simulink model "TV2016_CAN"  (Simulink 8.5)
settings: Solver=ode1  StartTime=0.0  StopTime=inf  FixedStep=0.001  RelTol=1e-3
PreLoadFcn:
  | FSE_Parameters
values from neighbouring files (symbols this model uses):
  car_params = Simulink_Car_params    [TV2016_parameters.m]
  i_Diff = 15.47    [TV2016_parameters.m]
  Kp = 1    [TV2016_parameters.m]
  settings = Simulink_Settings    [TV2016_parameters.m]
  SpdC_BCC = 0    [TV2016_parameters.m]
  Speed_Neg_sat = -21    [TV2016_parameters.m]
  Speed_Pos_sat = 21    [TV2016_parameters.m]
  Tn_n = 0    [TV2016_parameters.m]
  Use_Joystick = 1    [TV2016_parameters.m]
undefined symbols (not defined in the file or in its folder): canChannel
libraries: CarMaker4SL x139, simulink x18, canmsglib x10, simulink_extras x7, canlib x5, sldrtlib x1
(part 1 of 4)
settings Model: Creator=fh  LastModifiedBy=Will
settings SolverCC: EnableConcurrentExecution=on  InsertRTBMode=Always
settings DataIOCC: SignalLoggingName=sigsOut
settings OptimizationCC: BlockReduction=off  OptimizeBlockIOStorage=off  BufferReuse=off  GlobalBufferReuse=off  ExpressionFolding=off  LocalBlockOutputs=off  InitFltsAndDblsToZero=on
settings DebuggingCC: SaveWithParameterizedLinksMsg=none  SignalResolutionControl=TryResolveAllWithWarning  MultiTaskDSMMsg=warning  MultiTaskCondExecSysMsg=none  FcnCallInpInsideContextMsg=UseLocalSettings  BusObjectLabelMismatch=error
settings HardwareCC: ProdBitPerLong=64  ProdBitPerPointer=64  ProdIntDivRoundTo=Zero  ProdEndianess=LittleEndian  ProdWordSize=64  ProdHWDeviceType=Intel->x86-64  TargetBitPerLong=64  TargetBitPerPointer=64  TargetIntDivRoundTo=Zero  TargetEndianess=LittleEndian  TargetWordSize=64  TargetHWDeviceType=Intel->x86-64
settings SFSimCC: SimCtrlC=off
settings RTWCC: SystemTargetFile=rtwin.tlc  TemplateMakefile=rtwin.tmf  Description=Simulink Desktop Real-Time  Toolchain=LCC-win64 v2.4.1 | gmake (64-bit Windows)  BuildConfiguration=Faster Runs  RTWCompilerOptimization=on  CheckMdlBeforeBuild=Warning
settings CodeAppCC: MaxIdLength=95
settings RTWinTargetCC: TargetPreCompLibLocation=D:\Program Files\MATLAB\R2015a\toolbox\sldrt\lib\win64

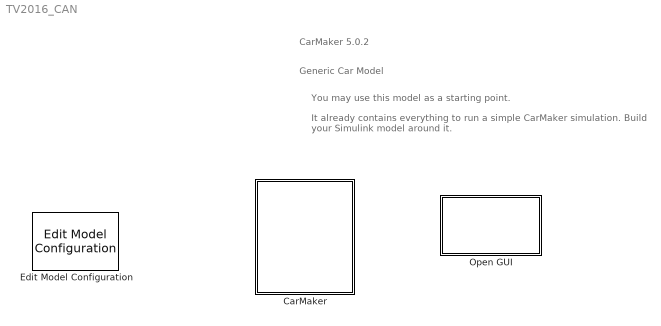
== system TV2016_CAN ==
  note: Generic Car Model
  note: You may use this model as a starting point.
  note: It already contains everything to run a simple CarMaker simulation.
      | Build your Simulink model around it.
  note: CarMaker 5.0.2
  CarMaker : Subsystem  TreatAsAtomicUnit=on
      mask Display: image(imread('CarMaker4SLss.bmp'));
  Edit Model Configuration : CarMaker4SL/Edit Model Configuration
  Open GUI : Subsystem  LoadFcn=if ~length(which('cmcmd')), cmenv; end
      settings: OpenFcn=cmblockmagic('gui_fix_display'); CM_Simulink
      mask Display: image(imread('CarMakerGUI.bmp'));

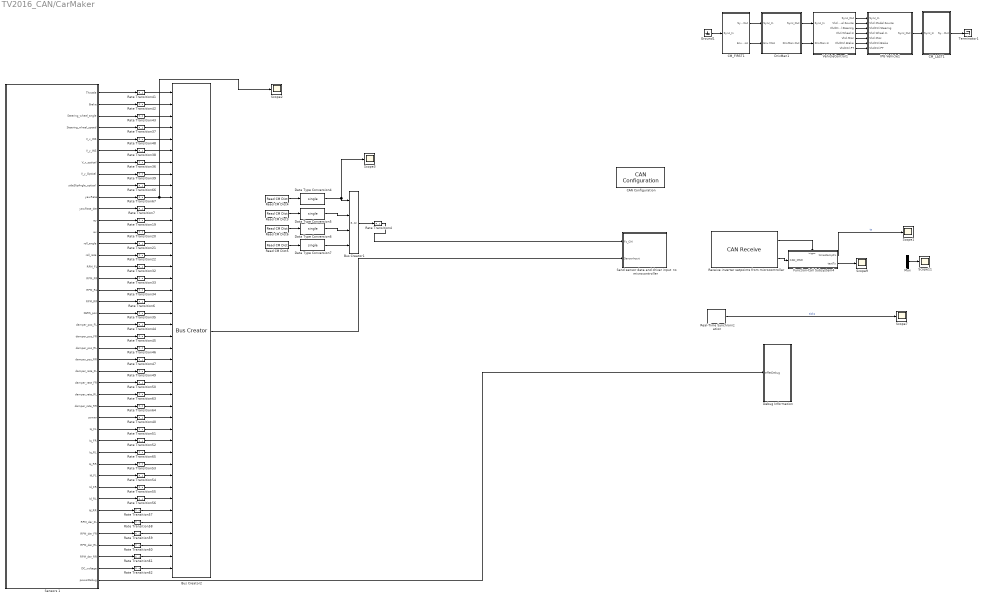
== system TV2016_CAN/CarMaker ==
  Bus Creator1 : BusCreator  OutDataTypeStr=Bus: normalForces  NonVirtualBus=on
      settings: InheritFromInputs=off
  Bus Creator2 : BusCreator  Inputs=42  OutDataTypeStr=Bus: SensorInputs  NonVirtualBus=on
      settings: InheritFromInputs=off
  CAN Configuration : canlib/CAN Configuration  BlockHandle=4619.0087  DeviceMenu=(none)  Device=PEAK-System PCAN-USB (PCAN_USBBUS1)  ObjConstructor=canChannel('PEAK-System', 'PCAN_USBBUS1')  BusSpeed=1000000  EnableBitParameters=off  SJW=NaN  TSEG1=NaN  TSEG2=NaN  NSamples=NaN  AckMode=Normal
  CM_FIRST1 : Subsystem
  CM_LAST1 : Subsystem
  Data Type Conversion{4..7} (4 alike) : DataTypeConversion  OutDataTypeStr=single
  "Debug Information " : Subsystem
  DrivMan1 : Subsystem
  Function-Call Subsystem4 : Subsystem  TreatAsAtomicUnit=on
  Ground1 : Ground
  IPG Vehicle1 : Subsystem  TreatAsAtomicUnit=on
  Mux : Mux  Inputs=2
  Rate Transition{4,6..7,19..22,32..67} (43 alike) : RateTransition  OutPortSampleTime=settings.sensor_sampling_time
  Read CM Dict3 : CarMaker4SL/Read CM Dict  xname=Vhcl.FR.Fz  xsync=off
  Read CM Dict4 : CarMaker4SL/Read CM Dict  xname=Vhcl.FL.Fz  xsync=off
  Read CM Dict5 : CarMaker4SL/Read CM Dict  xname=Vhcl.RR.Fz  xsync=off
  Read CM Dict6 : CarMaker4SL/Read CM Dict  xname=Vhcl.RL.Fz  xsync=off
  Real-Time Synchronization : sldrtlib/Real-Time Synchronization  SampleTime=0.001  MaxMissedTicks=100000  ShowMissedTicks=on  YieldWhenWaiting=off
  Receive inverter setpoints from microcontroller : canlib/CAN Receive  BlockHandle=12566.0002  DeviceMenu=(none)  Device=PEAK-System PCAN-USB (PCAN_USBBUS1)  ObjConstructor=canChannel('PEAK-System', 'PCAN_USBBUS1')  EnableStandardIDsFilter=off  StandardIDs=[387,388,389,390,800]  EnableExtendedIDsFilter=off  ExtendedIDs=0  SampleTime=0.001  MsgsPerTimestep=all  StdIDsCombo=Allow only  ExtIDsCombo=Block all  InternalFilterUpdateStatus=on
  Scope{1..3,7,9,11} (6 alike) : Scope
      Scope1 settings: ShowLegends=on  TimeRange=2.184524711696869  YMin=-0.01  YMax=0.02  SaveName=ScopeData26
      Scope11 settings: ShowLegends=on  TimeRange=2.184524711696869  YMin=-0.01  YMax=0.02  SaveName=ScopeData25
      Scope2 settings: ShowLegends=on  TimeRange=9.572585353545549e-05  YMin=0  YMax=1000  SaveName=ScopeData45
      Scope3 settings: ShowLegends=on  TimeRange=9.572585353545549e-05  YMin=0  YMax=1000  SaveName=ScopeData51
      Scope7 settings: ShowLegends=on  TimeRange=9.572585353545549e-05  YMin=0  YMax=1000  SaveName=ScopeData14
      Scope9 settings: YMin=2  YMax=15  SaveName=ScopeData38  SampleInput=on  SampleTime=0.001
  "Send sensor data and driver input  to microcontroller " : Subsystem
  Sensors 1 : Subsystem  SystemSampleTime=settings.control_system_sample_time
  Terminator1 : Terminator
  VehicleControl1 : Subsystem
  wires:
  Read CM Dict3/1 -> Data Type Conversion5/1
  Read CM Dict4/1 -> Data Type Conversion4/1
  Read CM Dict5/1 -> Data Type Conversion7/1
  Read CM Dict6/1 -> Data Type Conversion6/1
  Data Type Conversion6/1 -> Bus Creator1/3
  Data Type Conversion7/1 -> Bus Creator1/4
  Data Type Conversion5/1 -> Bus Creator1/2
  Data Type Conversion4/1 -> Scope3/1, Bus Creator1/1
  Bus Creator1/1 -> Rate Transition4/1
  Rate Transition4/1 -> "Send sensor data and driver input  to microcontroller "/1(Fz_CM)
  Real-Time Synchronization/1 -> Scope7/1  "ticks"
  Receive inverter setpoints from microcontroller/2 -> Function-Call Subsystem4/1(CAN_MSG)
  Receive inverter setpoints from microcontroller/1 -> Function-Call Subsystem4/Trigger
  Function-Call Subsystem4/1(timestampFL) -> Scope1/1  "ts"
  Mux/1 -> Scope11/1
  Function-Call Subsystem4/2(testTs) -> Scope9/1
  Sensors 1/43(powerDebug) -> "Debug Information "/1(effetDebug)
  Bus Creator2/1 -> "Send sensor data and driver input  to microcontroller "/2(SensorInput)
  Sensors 1/40(RPM_der_RL) -> Rate Transition60/1
  Sensors 1/41(RPM_der_RR) -> Rate Transition61/1
  Sensors 1/39(RPM_der_FR) -> Rate Transition59/1
  Sensors 1/38(RPM_der_FL) -> Rate Transition58/1
  Sensors 1/37(Id_RR) -> Rate Transition57/1
  Sensors 1/4(Steering_wheel_speed) -> Rate Transition37/1
  Sensors 1/1("Throttle ") -> Rate Transition41/1
  Sensors 1/2("Brake ") -> Rate Transition42/1
  Sensors 1/3("Steering_wheel_angle ") -> Rate Transition43/1
  Sensors 1/5(V_x_INS) -> Rate Transition48/1
  Sensors 1/6(V_y_INS) -> Rate Transition38/1
  Sensors 1/7(V_x_optical) -> Rate Transition36/1
  Sensors 1/8(V_y_Optical) -> Rate Transition39/1
  Sensors 1/9(sideSlipAngle_optical) -> Rate Transition66/1
  Sensors 1/10(yawRate) -> Rate Transition67/1
  Sensors 1/12(ay) -> Rate Transition19/1
  Sensors 1/13("ax ") -> Rate Transition20/1
  Sensors 1/14(roll_angle) -> Rate Transition21/1
  Sensors 1/15(roll_rate) -> Rate Transition22/1
  Sensors 1/16(RPM_FL) -> Rate Transition32/1
  Sensors 1/17(RPM_FR) -> Rate Transition33/1
  Sensors 1/18(RPM_RL) -> Rate Transition34/1
  Sensors 1/19(RPM_RR) -> Rate Transition6/1
  Sensors 1/20(KERS_pos) -> Rate Transition35/1
  Sensors 1/21(damper_pos_FL) -> Rate Transition44/1
  Sensors 1/22(damper_pos_FR) -> Rate Transition45/1
  Sensors 1/23(damper_pos_RL) -> Rate Transition46/1
  Sensors 1/24(damper_pos_RR) -> Rate Transition47/1
  Sensors 1/25(damper_rate_FL) -> Rate Transition49/1
  Sensors 1/26(damper_rate_FR) -> Rate Transition50/1
  Sensors 1/27(damper_rate_RL) -> Rate Transition63/1
  Sensors 1/28(damper_rate_RR) -> Rate Transition64/1
  Sensors 1/29(power) -> Rate Transition40/1
  Sensors 1/30(Iq_FL) -> Rate Transition51/1
  Sensors 1/31(Iq_FR) -> Rate Transition52/1
  Sensors 1/32(Iq_RL) -> Rate Transition65/1
  Sensors 1/33(Iq_RR) -> Rate Transition53/1
  Sensors 1/34(Id_FL) -> Rate Transition54/1
  Sensors 1/35(Id_FR) -> Rate Transition55/1
  Sensors 1/36(Id_RL) -> Rate Transition56/1
  Sensors 1/11(yawRate_der) -> Rate Transition7/1
  Sensors 1/42(DC_voltage) -> Rate Transition62/1
  Rate Transition62/1 -> Bus Creator2/42
  Rate Transition6/1 -> Bus Creator2/19
  Rate Transition7/1 -> Bus Creator2/11
  Rate Transition19/1 -> Bus Creator2/12
  Rate Transition20/1 -> Bus Creator2/13
  Rate Transition21/1 -> Bus Creator2/14
  Rate Transition22/1 -> Bus Creator2/15
  Rate Transition32/1 -> Bus Creator2/16
  Rate Transition33/1 -> Bus Creator2/17
  Rate Transition34/1 -> Bus Creator2/18
  Rate Transition35/1 -> Bus Creator2/20
  Rate Transition36/1 -> Bus Creator2/7
  Rate Transition37/1 -> Bus Creator2/4
  Rate Transition38/1 -> Bus Creator2/6
  Rate Transition39/1 -> Bus Creator2/8
  Rate Transition40/1 -> Bus Creator2/29
  Rate Transition41/1 -> Bus Creator2/1
  Rate Transition42/1 -> Bus Creator2/2
  Rate Transition43/1 -> Bus Creator2/3
  Rate Transition44/1 -> Bus Creator2/21
  Rate Transition45/1 -> Bus Creator2/22
  Rate Transition46/1 -> Bus Creator2/23
  Rate Transition47/1 -> Bus Creator2/24
  Rate Transition48/1 -> Bus Creator2/5
  Rate Transition49/1 -> Bus Creator2/25
  Rate Transition50/1 -> Bus Creator2/26
  Rate Transition51/1 -> Bus Creator2/30
  Rate Transition52/1 -> Bus Creator2/31
  Rate Transition53/1 -> Bus Creator2/33
  Rate Transition54/1 -> Bus Creator2/34
  Rate Transition55/1 -> Bus Creator2/35
  Rate Transition56/1 -> Bus Creator2/36
  Rate Transition63/1 -> Bus Creator2/27
  Rate Transition64/1 -> Bus Creator2/28
  Rate Transition65/1 -> Bus Creator2/32
  Rate Transition66/1 -> Bus Creator2/9
  Rate Transition67/1 -> Scope2/1, Bus Creator2/10
  Rate Transition57/1 -> Bus Creator2/37
  Rate Transition58/1 -> Bus Creator2/38
  Rate Transition59/1 -> Bus Creator2/39
  Rate Transition60/1 -> Bus Creator2/40
  Rate Transition61/1 -> Bus Creator2/41
  DrivMan1/2(DrivMan.Out) -> VehicleControl1/2(DrivMan.In)
  DrivMan1/1(Sync_Out) -> VehicleControl1/1(Sync_In)
  CM_FIRST1/2(Env.Misc) -> DrivMan1/2(Env.Misc)
  CM_FIRST1/1(Sync_Out) -> DrivMan1/1(Sync_In)
  CM_LAST1/1(Sync_Out) -> Terminator1/1
  IPG Vehicle1/1(Sync_Out) -> CM_LAST1/1(Sync_In)
  VehicleControl1/1(Sync_Out) -> IPG Vehicle1/1(Sync_In)
  VehicleControl1/3(VhclCtrl.Steering) -> IPG Vehicle1/3(VhclCtrl.Steering)
  VehicleControl1/4(Vhcl.Wheel.In) -> IPG Vehicle1/4(Vhcl.Wheel.In)
  VehicleControl1/5(Vhcl.Misc) -> IPG Vehicle1/5(Vhcl.Misc)
  VehicleControl1/6(VhclCtrl.Brake) -> IPG Vehicle1/6(VhclCtrl.Brake)
  VehicleControl1/7(VhclCtrl.PT) -> IPG Vehicle1/7(VhclCtrl.PT)
  VehicleControl1/2(Vhcl.Model.Source) -> IPG Vehicle1/2(Vhcl.Model.Source)
  Ground1/1 -> CM_FIRST1/1(Sync_In)

== system TV2016_CAN/Open GUI ==
  S-Function : S-Function  FunctionName=cm_gui

== system TV2016_CAN/CarMaker/CM_FIRST1 ==
  Sync_In : Inport
  Bus Creator1 : BusCreator  Inputs=9
  Demux : Demux  Outputs=9
  Environment : S-Function  FunctionName=CM_Sfun  Parameters='Environment'
  IoIn : S-Function  FunctionName=CM_Sfun  Parameters='IoIn'
  Sync_Out : Outport
  Env.Misc : Outport  Port=2
  wires:
  Bus Creator1/1 -> Env.Misc/1
  Environment/2 -> Demux/1
  Demux/4 -> Bus Creator1/4  "Env AirHumidity"
  Demux/3 -> Bus Creator1/3  "Env AirPressure"
  Demux/2 -> Bus Creator1/2  "Env AirDensity"
  Demux/1 -> Bus Creator1/1  "Env Temperature"
  Environment/1 -> Sync_Out/1
  IoIn/1 -> Environment/1
  Sync_In/1 -> IoIn/1
  Demux/5 -> Bus Creator1/5  "Env Time"
  Demux/6 -> Bus Creator1/6  "Env SolarRadiation"
  Demux/7 -> Bus Creator1/7  "Env WindVel_tot x"
  Demux/8 -> Bus Creator1/8  "Env WindVel_tot y"
  Demux/9 -> Bus Creator1/9  "Env WindVel_tot z"

== system TV2016_CAN/CarMaker/CM_LAST1 ==
  Sync_In : Inport
  CM_User : S-Function  FunctionName=CM_Sfun  Parameters='CM_User'
  IoOut : S-Function  FunctionName=CM_Sfun  Parameters='IoOut'
  Sync_Out : Outport
  wires:
  IoOut/1 -> Sync_Out/1
  CM_User/1 -> IoOut/1
  Sync_In/1 -> CM_User/1

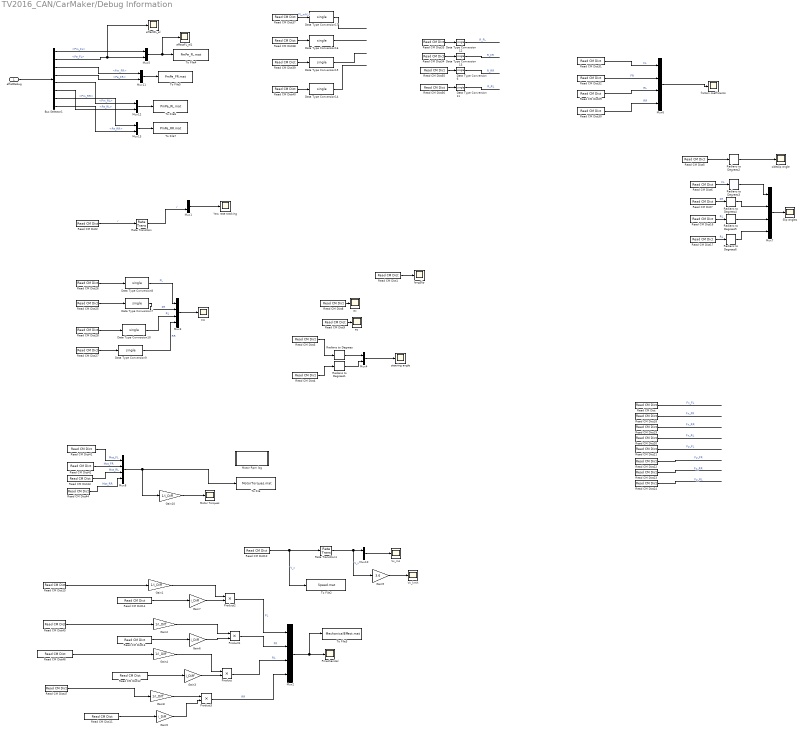
== system TV2016_CAN/CarMaker/Debug Information  ==
  effetDebug : Inport
  Bus Selector1 : BusSelector  OutputSignals=Pm_FL,Pe_FL,Pm_FR,Pe_FR,Pm_RL,Pe_RL,Pm_RR,Pe_RR
  Data Type Conversion{6..17} (12 alike) : DataTypeConversion  OutDataTypeStr=single
  Fzi : Scope
      settings: ShowLegends=on  TimeRange=18.75514233997038  YMin=0  YMax=1400  SaveName=ScopeData21
  Gain{1..2,4,8,10} (5 alike) : Gain  Gain=1/i_Diff
  Gain{3,5..7} (4 alike) : Gain  Gain=i_Diff
  Gain9 : Gain  Gain=3.6
  "Motor Rpm log  " : Subsystem
  "Motor Torques " : Scope
      settings: ShowLegends=on  TimeRange=0.2362659824329911  YMin=0.3167539267015711  YMax=0.6151832460732987  SaveName=ScopeData8
  Mux{1,4..5,10..13} (7 alike) : Mux  Inputs=2
  Mux{2..3,6..8} (5 alike) : Mux
  Pmechanical : Scope
      settings: TimeRange=6  YMin=-25  YMax=275  SaveName=ScopeData20
  Product{,1..3} (4 alike) : Product
  Radians to Degrees{,1..6} (7 alike) : simulink_extras/Transformations/Radians to Degrees
  Rate Transition : RateTransition  OutPortSampleTime=settings.control_system_sample_time
  Rate Transition1 : RateTransition  OutPortSampleTime=settings.control_system_sample_time
  Read CM Dict : CarMaker4SL/Read CM Dict  xname=Vhcl.FL.Fx  xsync=off
  Read CM Dict1 : CarMaker4SL/Read CM Dict  xname=Car.LongSlipRL  xsync=off
  Read CM Dict10 : CarMaker4SL/Read CM Dict  xname=Car.vx  xsync=off
  Read CM Dict11 : CarMaker4SL/Read CM Dict  xname=Car.WheelSpd_RR  xsync=off
  Read CM Dict12 : CarMaker4SL/Read CM Dict  xname=Car.WheelSpd_RL  xsync=off
  Read CM Dict13 : CarMaker4SL/Read CM Dict  xname=Car.WheelSpd_FR  xsync=off
  Read CM Dict14 : CarMaker4SL/Read CM Dict  xname=Car.WheelSpd_FL  xsync=off
  Read CM Dict15 : CarMaker4SL/Read CM Dict  xname=PT.WFL.Trq_Drive  xsync=off
  Read CM Dict16 : CarMaker4SL/Read CM Dict  xname=Car.SlipAngleRL  xsync=off
  Read CM Dict17 : CarMaker4SL/Read CM Dict  xname=Car.SlipAngleRR  xsync=off
  Read CM Dict18 : CarMaker4SL/Read CM Dict  xname=Vhcl.FR.Fx  xsync=off
  Read CM Dict19 : CarMaker4SL/Read CM Dict  xname=Vhcl.RR.Fx  xsync=off
  Read CM Dict2 : CarMaker4SL/Read CM Dict  xname=Car.YawRate  xsync=off
  Read CM Dict20 : CarMaker4SL/Read CM Dict  xname=Vhcl.RL.Fx  xsync=off
  Read CM Dict21 : CarMaker4SL/Read CM Dict  xname=Vhcl.FL.Fy  xsync=off
  Read CM Dict22 : CarMaker4SL/Read CM Dict  xname=Vhcl.FR.Fy  xsync=off
  Read CM Dict23 : CarMaker4SL/Read CM Dict  xname=Vhcl.RR.Fy  xsync=off
  Read CM Dict24 : CarMaker4SL/Read CM Dict  xname=Vhcl.RL.Fy  xsync=off
  Read CM Dict25 : CarMaker4SL/Read CM Dict  xname=Vhcl.FR.Fz  xsync=off
  Read CM Dict26 : CarMaker4SL/Read CM Dict  xname=Vhcl.FL.Fz  xsync=off
  Read CM Dict27 : CarMaker4SL/Read CM Dict  xname=Vhcl.RR.Fz  xsync=off
  Read CM Dict28 : CarMaker4SL/Read CM Dict  xname=Vhcl.RL.Fz  xsync=off
  Read CM Dict29 : CarMaker4SL/Read CM Dict  xname=Car.muRoadRL  xsync=off
  Read CM Dict3 : CarMaker4SL/Read CM Dict  xname=Car.CFR.rz  xsync=off
  Read CM Dict30 : CarMaker4SL/Read CM Dict  xname=Car.muRoadRR  xsync=off
  Read CM Dict31 : CarMaker4SL/Read CM Dict  xname=Car.muRoadFL  xsync=off
  Read CM Dict32 : CarMaker4SL/Read CM Dict  xname=Car.muRoadFR  xsync=off
  Read CM Dict33 : CarMaker4SL/Read CM Dict  xname=Car.WFL.Radius  xsync=off
  Read CM Dict34 : CarMaker4SL/Read CM Dict  xname=Car.WFR.Radius  xsync=off
  Read CM Dict35 : CarMaker4SL/Read CM Dict  xname=Car.WRR.Radius  xsync=off
  Read CM Dict36 : CarMaker4SL/Read CM Dict  xname=Car.WRL.Radius  xsync=off
  Read CM Dict37 : CarMaker4SL/Read CM Dict  xname=Car.vFL  xsync=off
  Read CM Dict38 : CarMaker4SL/Read CM Dict  xname=Car.vFR  xsync=off
  Read CM Dict39 : CarMaker4SL/Read CM Dict  xname=Car.vRR  xsync=off
  Read CM Dict4 : CarMaker4SL/Read CM Dict  xname=Car.CFL.rz  xsync=off
  Read CM Dict40 : CarMaker4SL/Read CM Dict  xname=Car.vRL  xsync=off
  Read CM Dict41 : CarMaker4SL/Read CM Dict  xname=PT.WFL.Trq_Drive  xsync=off
  Read CM Dict42 : CarMaker4SL/Read CM Dict  xname=PT.WFR.Trq_Drive  xsync=off
  Read CM Dict43 : CarMaker4SL/Read CM Dict  xname=PT.WRL.Trq_Drive  xsync=off
  Read CM Dict44 : CarMaker4SL/Read CM Dict  xname=PT.WRR.Trq_Drive  xsync=off
  Read CM Dict45 : CarMaker4SL/Read CM Dict  xname=PT.WFR.Trq_Drive  xsync=off
  Read CM Dict46 : CarMaker4SL/Read CM Dict  xname=PT.WRL.Trq_Drive  xsync=off
  Read CM Dict47 : CarMaker4SL/Read CM Dict  xname=PT.WRR.Trq_Drive  xsync=off
  Read CM Dict5 : CarMaker4SL/Read CM Dict  xname=Car.SideSlipAngle  xsync=off
  Read CM Dict6 : CarMaker4SL/Read CM Dict  xname=Car.SlipAngleFL  xsync=off
  Read CM Dict7 : CarMaker4SL/Read CM Dict  xname=Car.SlipAngleFR  xsync=off
  Read CM Dict8 : CarMaker4SL/Read CM Dict  xname=Car.ax  xsync=off
  Read CM Dict9 : CarMaker4SL/Read CM Dict  xname=Car.ay  xsync=off
  Slip angles : Scope
      settings: YMin=-0.025  YMax=0.325  SaveName=ScopeData24
  To File : ToFile  Filename=MotorTorques.mat  MatrixName=MotorTorques  SaveFormat=Timeseries
  To File2 : ToFile  Filename=Speed.mat  MatrixName=VehicleSpeed  SaveFormat=Timeseries
  To File3 : ToFile  Filename=MechanicalEffect.mat  MatrixName=MechEffect  SaveFormat=Timeseries
  To File4 : ToFile  Filename=PmPe_FL.mat  MatrixName=PmPe_FL  SaveFormat=Timeseries
  To File5 : ToFile  Filename=PmPe_FR.mat  MatrixName=PmPe_FR  SaveFormat=Timeseries
  To File6 : ToFile  Filename=PmPe_RL.mat  MatrixName=PmPe_RL  SaveFormat=Timeseries
  To File7 : ToFile  Filename=PmPe_RR.mat  MatrixName=PmPe_RR  SaveFormat=Timeseries
  Vx_kmh : Scope
      settings: ShowLegends=on  TimeRange=0.02126907879490897  YMin=71.75  YMax=75.25  SaveName=ScopeData27
  "Vx_ms " : Scope
      settings: ShowLegends=on  TimeRange=0.02126907879490897  YMin=0  YMax=35  SaveName=ScopeData15
  Yaw rate tracking : Scope
      settings: ShowLegends=on  TimeRange=51.98675496688742  YMin=-0.4  YMax=0.9  SaveName=ScopeData5
  ax : Scope
      settings: YMin=-0.025  YMax=0.325  SaveName=ScopeData11
  ay : Scope
      settings: YMin=-15  YMax=12.5  SaveName=ScopeData12
  effectFL_el : Scope
      settings: ShowLegends=on  TimeRange=51.98675496688742  YMin=-1.5  YMax=1.5  SaveName=ScopeData19
  effectFL_el1 : Scope
      settings: ShowLegends=on  TimeRange=51.98675496688742  YMin=-1.5  YMax=1.5  SaveName=ScopeData33
  friction coefficients : Scope
      settings: YMin=-0.04  YMax=0.055
  "longSlip " : Scope
      settings: YMin=-0.025  YMax=0.325  SaveName=ScopeData4
  sideslip angle : Scope
      settings: YMin=-0.04  YMax=0.055  SaveName=ScopeData22
  steering angle : Scope
      settings: ShowLegends=on  TimeRange=0.06245515784438777  YMin=-26.5  YMax=-21.5  SaveName=ScopeData17
  wires:
  Read CM Dict8/1 -> ax/1
  Read CM Dict9/1 -> ay/1
  Read CM Dict10/1 -> Rate Transition1/1, To File2/1  "V_x"
  Mux4/1 -> steering angle/1
  Read CM Dict3/1 -> Radians to Degrees/1
  Read CM Dict4/1 -> Radians to Degrees1/1
  Radians to Degrees/1 -> Mux4/1
  Radians to Degrees1/1 -> Mux4/2
  Read CM Dict1/1 -> "longSlip "/1
  Read CM Dict2/1 -> Rate Transition/1  "r"
  Mux1/1 -> Yaw rate tracking/1
  Read CM Dict5/1 -> Radians to Degrees2/1
  Read CM Dict6/1 -> Radians to Degrees3/1  "FL"
  Read CM Dict7/1 -> Radians to Degrees4/1  "FR"
  Read CM Dict16/1 -> Radians to Degrees5/1  "RL"
  Read CM Dict17/1 -> Radians to Degrees6/1  "RL"
  Mux7/1 -> Slip angles/1
  Radians to Degrees2/1 -> sideslip angle/1
  Radians to Degrees3/1 -> Mux7/1
  Radians to Degrees4/1 -> Mux7/2
  Radians to Degrees5/1 -> Mux7/3
  Radians to Degrees6/1 -> Mux7/4
  Read CM Dict18/1 -> ?  "Fx_FR"
  Read CM Dict20/1 -> ?  "Fx_RL"
  Read CM Dict19/1 -> ?  "Fx_RR"
  Read CM Dict/1 -> ?  "Fx_FL"
  Read CM Dict21/1 -> ?  "Fy_FL"
  Read CM Dict23/1 -> ?  "Fy_RR"
  Read CM Dict24/1 -> ?  "Fy_RL"
  Read CM Dict22/1 -> ?  "Fy_FR"
  Read CM Dict25/1 -> Data Type Conversion7/1
  Read CM Dict28/1 -> Data Type Conversion10/1
  Data Type Conversion10/1 -> Mux3/3  "RL"
  Data Type Conversion7/1 -> Mux3/2  "FR"
  Mux3/1 -> Fzi/1
  Read CM Dict26/1 -> Data Type Conversion8/1
  Data Type Conversion8/1 -> Mux3/1  "FL"
  Read CM Dict27/1 -> Data Type Conversion9/1
  Data Type Conversion9/1 -> Mux3/4  "RR"
  Mux6/1 -> friction coefficients/1
  Read CM Dict32/1 -> Mux6/2  "FR"
  Read CM Dict29/1 -> Mux6/3  "RL"
  Read CM Dict31/1 -> Mux6/1  "FL"
  Read CM Dict30/1 -> Mux6/4  "RR"
  Read CM Dict33/1 -> Data Type Conversion12/1
  Read CM Dict35/1 -> Data Type Conversion6/1
  Read CM Dict36/1 -> Data Type Conversion11/1
  Read CM Dict34/1 -> Data Type Conversion13/1
  Data Type Conversion11/1 -> ?  "R_RL"
  Data Type Conversion13/1 -> ?  "R_FR"
  Data Type Conversion6/1 -> ?  "R_RR"
  Data Type Conversion12/1 -> ?  "R_FL"
  Read CM Dict40/1 -> Data Type Conversion14/1
  Read CM Dict38/1 -> Data Type Conversion16/1
  Read CM Dict39/1 -> Data Type Conversion15/1
  Read CM Dict37/1 -> Data Type Conversion17/1  "FL_whl_v"
  Data Type Conversion17/1 -> ?
  Data Type Conversion16/1 -> ?
  Data Type Conversion15/1 -> ?
  Data Type Conversion14/1 -> ?
  Read CM Dict42/1 -> Mux8/2  "Mot_FR"
  Read CM Dict43/1 -> Mux8/3  "Mot_RL"
  Read CM Dict41/1 -> Mux8/1  "Mot_FL"
  Read CM Dict44/1 -> Mux8/4  "Mot_RR"
  Mux8/1 -> To File/1, Gain10/1
  Rate Transition/1 -> Mux1/2  "r"
  Read CM Dict12/1 -> Gain3/1
  Read CM Dict11/1 -> Gain5/1
  Read CM Dict13/1 -> Gain6/1
  Read CM Dict14/1 -> Gain7/1
  Gain3/1 -> Product/2
  Gain7/1 -> Product2/2
  Read CM Dict15/1 -> Gain1/1
  Gain6/1 -> Product1/2
  Read CM Dict45/1 -> Gain2/1
  Gain5/1 -> Product3/2
  Read CM Dict47/1 -> Gain8/1
  Product3/1 -> Mux2/4  "RR"
  Read CM Dict46/1 -> Gain4/1
  Product/1 -> Mux2/3  "RL"
  Product1/1 -> Mux2/2  "FR"
  Product2/1 -> Mux2/1  "FL"
  Mux2/1 -> To File3/1, Pmechanical/1
  Gain1/1 -> Product2/1
  Gain2/1 -> Product1/1
  Gain4/1 -> Product/1
  Gain8/1 -> Product3/1
  Mux10/1 -> "Vx_ms "/1
  Rate Transition1/1 -> Gain9/1, Mux10/1  "V_x"
  Gain9/1 -> Vx_kmh/1
  Mux5/1 -> effectFL_el1/1, To File4/1
  Mux11/1 -> To File5/1
  Mux12/1 -> To File6/1
  Mux13/1 -> To File7/1
  effetDebug/1 -> Bus Selector1/1
  Bus Selector1/1 -> Mux5/1  "<Pm_FL>"
  Bus Selector1/2 -> effectFL_el/1, Mux5/2  "<Pe_FL>"
  Bus Selector1/3 -> Mux11/1  "<Pm_FR>"
  Bus Selector1/4 -> Mux11/2  "<Pe_FR>"
  Bus Selector1/5 -> Mux12/1  "<Pm_RL>"
  Bus Selector1/6 -> Mux12/2  "<Pe_RL>"
  Bus Selector1/7 -> Mux13/1  "<Pm_RR>"
  Bus Selector1/8 -> Mux13/2  "<Pe_RR>"
  Gain10/1 -> "Motor Torques "/1

== system TV2016_CAN/CarMaker/DrivMan1 ==
  note: There's rarely a reason to override DrivMan signals.
      | Use the VehicleControl interface for this purpose.
  Sync_In : Inport
  Env.Misc : Inport  Port=2
  BusCreator : BusCreator  Inputs=17
  Demux : Demux  Outputs=17
  DrivMan : S-Function  FunctionName=CM_Sfun  Parameters='DrivMan'
  Sync_Out : Outport
  DrivMan.Out : Outport  Port=2
  wires:
  Demux/17 -> BusCreator/17  "DrivMan Steering Trq"
  Demux/16 -> BusCreator/16  "DrivMan Steering AngAcc"
  Demux/15 -> BusCreator/15  "DrivMan Steering AngVel"
  Demux/14 -> BusCreator/14  "DrivMan Steering Ang"
  Demux/13 -> BusCreator/13  "DrivMan Gas"
  Demux/12 -> BusCreator/12  "DrivMan Clutch"
  Demux/11 -> BusCreator/11  "DrivMan BrakePark"
  Demux/10 -> BusCreator/10  "DrivMan Brake"
  Demux/9 -> BusCreator/9  "DrivMan GearNo"
  Demux/8 -> BusCreator/8  "DrivMan SelectorCtrl"
  Demux/7 -> BusCreator/7  "DrivMan UserSignal4"
  Demux/6 -> BusCreator/6  "DrivMan UserSignal3"
  Demux/5 -> BusCreator/5  "DrivMan UserSignal2"
  Demux/4 -> BusCreator/4  "DrivMan UserSignal1"
  Demux/3 -> BusCreator/3  "DrivMan UserSignal0"
  Demux/2 -> BusCreator/2  "DrivMan Key"
  Demux/1 -> BusCreator/1  "DrivMan SST"
  Env.Misc/1 -> DrivMan/2
  Sync_In/1 -> DrivMan/1
  DrivMan/1 -> Sync_Out/1
  BusCreator/1 -> DrivMan.Out/1
  DrivMan/2 -> Demux/1

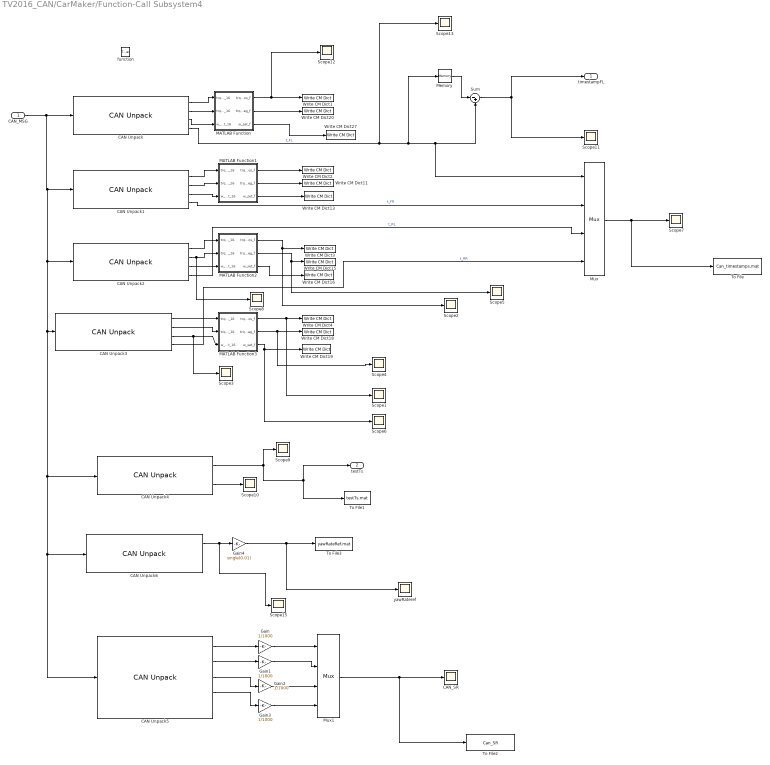
== system TV2016_CAN/CarMaker/Function-Call Subsystem4 ==
  CAN_MSG : Inport
  function : TriggerPort  TriggerType=function-call
  CAN Unpack : canmsglib/CAN Unpack  MsgList=(none)  MsgName=INV_FL  MsgIDType=Standard (11-bit identifier)  MsgIdentifier=387  MsgLength=6  SignalInfo=trq_pos$0$16$1$1$1$0$1$0$-Inf$Inf$#trq_neg$16$16$1$1$1$0$1$0$-Inf$Inf$#w_set$32$16$1$1$1$0$1$0$-Inf$Inf$#  NSignals=3  IDPort=off  TimestampPort=on  ErrorPort=off  RemotePort=off  LengthPort=off  StatusPort=off  StartBits=str2num('[int32(0);int32(16);int32(32)]')  SignalSizes=str2num('[int32(16);int32(16);int32(16)]')  ByteOrders=str2num('[int32(1);int32(1);int32(1)]')  DataTypes=str2num('[int32(1);int32(1);int32(1)]')  MultiplexTypes=str2num('[int32(1);int32(1);int32(1)]')  MultiplexValues=str2num('[double(0);double(0);double(0)]')  Factors=str2num('[double(1);double(1);double(1)]')  Offsets=str2num('[double(0);double(0);double(0)]')  Minimums=str2num('[double(-Inf);double(-Inf);double(-Inf)]')  Maximums=str2num('[double(Inf);double(Inf);double(Inf)]')
  CAN Unpack1 : canmsglib/CAN Unpack  MsgList=(none)  MsgName=INV_FR  MsgIDType=Standard (11-bit identifier)  MsgIdentifier=388  MsgLength=6  SignalInfo=trq_pos$0$16$1$1$1$0$1$0$-Inf$Inf$#trq_neg$16$16$1$1$1$0$1$0$-Inf$Inf$#w_set$32$16$1$1$1$0$1$0$-Inf$Inf$#  NSignals=3  IDPort=off  TimestampPort=on  ErrorPort=off  RemotePort=off  LengthPort=off  StatusPort=off  StartBits=str2num('[int32(0);int32(16);int32(32)]')  SignalSizes=str2num('[int32(16);int32(16);int32(16)]')  ByteOrders=str2num('[int32(1);int32(1);int32(1)]')  DataTypes=str2num('[int32(1);int32(1);int32(1)]')  MultiplexTypes=str2num('[int32(1);int32(1);int32(1)]')  MultiplexValues=str2num('[double(0);double(0);double(0)]')  Factors=str2num('[double(1);double(1);double(1)]')  Offsets=str2num('[double(0);double(0);double(0)]')  Minimums=str2num('[double(-Inf);double(-Inf);double(-Inf)]')  Maximums=str2num('[double(Inf);double(Inf);double(Inf)]')
  CAN Unpack2 : canmsglib/CAN Unpack  MsgList=(none)  MsgName=INV_RL  MsgIDType=Standard (11-bit identifier)  MsgIdentifier=389  MsgLength=6  SignalInfo=trq_pos$0$16$1$1$1$0$1$0$-Inf$Inf$#trq_neg$16$16$1$1$1$0$1$0$-Inf$Inf$#w_set$32$16$1$1$1$0$1$0$-Inf$Inf$#  NSignals=3  IDPort=off  TimestampPort=on  ErrorPort=off  RemotePort=off  LengthPort=off  StatusPort=off  StartBits=str2num('[int32(0);int32(16);int32(32)]')  SignalSizes=str2num('[int32(16);int32(16);int32(16)]')  ByteOrders=str2num('[int32(1);int32(1);int32(1)]')  DataTypes=str2num('[int32(1);int32(1);int32(1)]')  MultiplexTypes=str2num('[int32(1);int32(1);int32(1)]')  MultiplexValues=str2num('[double(0);double(0);double(0)]')  Factors=str2num('[double(1);double(1);double(1)]')  Offsets=str2num('[double(0);double(0);double(0)]')  Minimums=str2num('[double(-Inf);double(-Inf);double(-Inf)]')  Maximums=str2num('[double(Inf);double(Inf);double(Inf)]')
  CAN Unpack3 : canmsglib/CAN Unpack  MsgList=(none)  MsgName=INV_RR  MsgIDType=Standard (11-bit identifier)  MsgIdentifier=390  MsgLength=6  SignalInfo=trq_pos$0$16$1$1$1$0$1$0$-Inf$Inf$#trq_neg$16$16$1$1$1$0$1$0$-Inf$Inf$#w_set$32$16$1$1$1$0$1$0$-Inf$Inf$#  NSignals=3  IDPort=off  TimestampPort=on  ErrorPort=off  RemotePort=off  LengthPort=off  StatusPort=off  StartBits=str2num('[int32(0);int32(16);int32(32)]')  SignalSizes=str2num('[int32(16);int32(16);int32(16)]')  ByteOrders=str2num('[int32(1);int32(1);int32(1)]')  DataTypes=str2num('[int32(1);int32(1);int32(1)]')  MultiplexTypes=str2num('[int32(1);int32(1);int32(1)]')  MultiplexValues=str2num('[double(0);double(0);double(0)]')  Factors=str2num('[double(1);double(1);double(1)]')  Offsets=str2num('[double(0);double(0);double(0)]')  Minimums=str2num('[double(-Inf);double(-Inf);double(-Inf)]')  Maximums=str2num('[double(Inf);double(Inf);double(Inf)]')
  CAN Unpack4 : canmsglib/CAN Unpack  MsgList=(none)  MsgName=TestTimestamp  MsgIDType=Standard (11-bit identifier)  MsgIdentifier=800  MsgLength=4  SignalInfo=timestamp$0$32$1$2$1$0$1$0$-Inf$Inf$#  NSignals=1  IDPort=off  TimestampPort=on  ErrorPort=off  RemotePort=off  LengthPort=off  StatusPort=off  StartBits=str2num('[int32(0)]')  SignalSizes=str2num('[int32(32)]')  ByteOrders=str2num('[int32(1)]')  DataTypes=str2num('[int32(2)]')  MultiplexTypes=str2num('[int32(1)]')  MultiplexValues=str2num('[double(0)]')  Factors=str2num('[double(1)]')  Offsets=str2num('[double(0)]')  Minimums=str2num('[double(-Inf)]')  Maximums=str2num('[double(Inf)]')
  CAN Unpack5 : canmsglib/CAN Unpack  MsgList=(none)  MsgName=SlipRatios  MsgIDType=Standard (11-bit identifier)  MsgIdentifier=200  MsgLength=8  SignalInfo=SR_FL$0$16$1$1$1$0$1$0$-Inf$Inf$#SR_FR$16$16$1$1$1$0$1$0$-Inf$Inf$#SR_RL$32$16$1$1$1$0$1$0$-Inf$Inf$#SR_RR$48$16$1$1$1$0$1$0$-Inf$Inf$#  NSignals=4  IDPort=off  TimestampPort=on  ErrorPort=off  RemotePort=off  LengthPort=off  StatusPort=off  StartBits=str2num('[int32(0);int32(16);int32(32);int32(48)]')  SignalSizes=str2num('[int32(16);int32(16);int32(16);int32(16)]')  ByteOrders=str2num('[int32(1);int32(1);int32(1);int32(1)]')  DataTypes=str2num('[int32(1);int32(1);int32(1);int32(1)]')  MultiplexTypes=str2num('[int32(1);int32(1);int32(1);int32(1)]')  MultiplexValues=str2num('[double(0);double(0);double(0);double(0)]')  Factors=str2num('[double(1);double(1);double(1);double(1)]')  Offsets=str2num('[double(0);double(0);double(0);double(0)]')  Minimums=str2num('[double(-Inf);double(-Inf);double(-Inf);double(-Inf)]')  Maximums=str2num('[double(Inf);double(Inf);double(Inf);double(Inf)]')
  CAN Unpack6 : canmsglib/CAN Unpack  MsgList=(none)  MsgName=yawRatefeed  MsgIDType=Standard (11-bit identifier)  MsgIdentifier=201  MsgLength=2  SignalInfo=yawRate$0$16$1$1$1$0$1$0$-Inf$Inf$#  NSignals=1  IDPort=off  TimestampPort=on  ErrorPort=off  RemotePort=off  LengthPort=off  StatusPort=off  StartBits=str2num('[int32(0)]')  SignalSizes=str2num('[int32(16)]')  ByteOrders=str2num('[int32(1)]')  DataTypes=str2num('[int32(1)]')  MultiplexTypes=str2num('[int32(1)]')  MultiplexValues=str2num('[double(0)]')  Factors=str2num('[double(1)]')  Offsets=str2num('[double(0)]')  Minimums=str2num('[double(-Inf)]')  Maximums=str2num('[double(Inf)]')
  CAN_SR : Scope
      settings: ShowLegends=on  TimeRange=30  YMin=1785  YMax=1788.75  SaveName=ScopeData37  SampleInput=on
  Gain{,1..3} (4 alike) : Gain  Gain=1/1000
  Gain4 : Gain  Gain=single(0.01)
  MATLAB Function : MATLAB Function  TreatAsAtomicUnit=on
  MATLAB Function1 : MATLAB Function  TreatAsAtomicUnit=on
  MATLAB Function2 : MATLAB Function  TreatAsAtomicUnit=on
  MATLAB Function3 : MATLAB Function  TreatAsAtomicUnit=on
  Memory : Memory  InheritSampleTime=on
  Mux : Mux
  Mux1 : Mux
  Scope{1..13,15} (14 alike) : Scope
      Scope1 settings: YMin=0  YMax=11
      Scope10 settings: TimeRange=10  YMin=523.5  YMax=528.5  SaveName=ScopeData18
      Scope11 settings: ShowLegends=on  TimeRange=2.184524711696869  YMin=0.005  YMax=0.02  SaveName=ScopeData36  SampleInput=on
      Scope12 settings: ShowLegends=on  TimeRange=2.184524711696869  YMin=3.325  YMax=3.675  SaveName=ScopeData41  SampleInput=on
      Scope13 settings: ShowLegends=on  TimeRange=2.184524711696869  YMin=1460.25  YMax=1462.75  SaveName=ScopeData44  SampleInput=on
      Scope15 settings: TimeRange=10  YMin=523.5  YMax=528.5  SaveName=ScopeData49
      Scope2 settings: YMin=0  YMax=4.25
      Scope3 settings: YMin=-33196.8  YMax=30000  SaveName=ScopeData7
      Scope4 settings: YMin=0  YMax=11  SaveName=ScopeData2
      Scope5 settings: YMin=0  YMax=14  SaveName=ScopeData3
      Scope6 settings: TimeRange=10  YMin=0  YMax=11  SaveName=ScopeData6
      Scope7 settings: ShowLegends=on  TimeRange=30  YMin=1785  YMax=1788.75  SaveName=ScopeData9  SampleInput=on
      Scope8 settings: YMin=-9000  YMax=0  SaveName=ScopeData13
      Scope9 settings: YMin=2  YMax=15  SaveName=ScopeData16  SampleInput=on
  Sum : Sum  Inputs=|-+
  To File : ToFile  Filename=Can_timestamps.mat  MatrixName=ts  SaveFormat=Timeseries
  To File1 : ToFile  Filename=testTs.mat  MatrixName=testTs
  To File2 : ToFile  Filename=Can_SR  MatrixName=sr  SaveFormat=Timeseries
  To File3 : ToFile  Filename=yawRateRef.mat  MatrixName=rRef  SaveFormat=Timeseries
  Write CM Dict1 : CarMaker4SL/Write CM Dict  xname=Tlim_pos_FL  xsync=off
  Write CM Dict11 : CarMaker4SL/Write CM Dict  xname=Tlim_neg_FR  xsync=off
  Write CM Dict13 : CarMaker4SL/Write CM Dict  xname=w_set_FR  xsync=off
  Write CM Dict15 : CarMaker4SL/Write CM Dict  xname=Tlim_neg_RL  xsync=off
  Write CM Dict16 : CarMaker4SL/Write CM Dict  xname=w_set_RL  xsync=off
  Write CM Dict18 : CarMaker4SL/Write CM Dict  xname=Tlim_neg_RR  xsync=off
  Write CM Dict19 : CarMaker4SL/Write CM Dict  xname=w_set_RR  xsync=off
  Write CM Dict2 : CarMaker4SL/Write CM Dict  xname=Tlim_pos_FR  xsync=off
  Write CM Dict20 : CarMaker4SL/Write CM Dict  xname=Tlim_neg_FL  xsync=off
  Write CM Dict27 : CarMaker4SL/Write CM Dict  xname=w_set_FL  xsync=off
  Write CM Dict3 : CarMaker4SL/Write CM Dict  xname=Tlim_pos_RL  xsync=off
  Write CM Dict4 : CarMaker4SL/Write CM Dict  xname=Tlim_pos_RR  xsync=off
  yawRateref : Scope
      settings: TimeRange=10  YMin=523.5  YMax=528.5  SaveName=ScopeData48
  timestampFL : Outport
  testTs : Outport  Port=2
  wires:
  CAN_MSG/1 -> CAN Unpack2/1, CAN Unpack6/1, CAN Unpack5/1, CAN Unpack4/1, CAN Unpack3/1, CAN Unpack1/1, CAN Unpack/1
  CAN Unpack/2 -> MATLAB Function/2(trq_neg_16)
  CAN Unpack/3 -> MATLAB Function/3(w_set_16)
  CAN Unpack/1 -> MATLAB Function/1(trq_pos_16)
  MATLAB Function/1(trq_pos_f) -> Scope12/1, Write CM Dict1/1
  MATLAB Function/2(trq_neg_f) -> Write CM Dict20/1
  MATLAB Function/3(w_set_f) -> Write CM Dict27/1
  CAN Unpack1/2 -> MATLAB Function1/2(trq_neg_16)
  CAN Unpack1/1 -> MATLAB Function1/1(trq_pos_16)
  CAN Unpack1/3 -> MATLAB Function1/3(w_set_16)
  MATLAB Function1/1(trq_pos_f) -> Write CM Dict2/1
  MATLAB Function1/2(trq_neg_f) -> Write CM Dict11/1
  MATLAB Function1/3(w_set_f) -> Write CM Dict13/1
  CAN Unpack2/1 -> MATLAB Function2/1(trq_pos_16)
  CAN Unpack2/2 -> MATLAB Function2/2(trq_neg_16), Scope8/1
  CAN Unpack2/3 -> MATLAB Function2/3(w_set_16)
  MATLAB Function2/3(w_set_f) -> Write CM Dict16/1
  MATLAB Function2/2(trq_neg_f) -> Scope5/1, Write CM Dict15/1
  MATLAB Function2/1(trq_pos_f) -> Scope2/1, Write CM Dict3/1
  CAN Unpack3/1 -> MATLAB Function3/1(trq_pos_16)
  CAN Unpack3/2 -> MATLAB Function3/2(trq_neg_16)
  CAN Unpack3/3 -> MATLAB Function3/3(w_set_16), Scope3/1
  MATLAB Function3/3(w_set_f) -> Scope6/1, Write CM Dict19/1
  MATLAB Function3/2(trq_neg_f) -> Scope4/1, Write CM Dict18/1
  MATLAB Function3/1(trq_pos_f) -> Scope1/1, Write CM Dict4/1
  CAN Unpack2/4 -> Mux/3  "t_RL"
  CAN Unpack/4 -> Memory/1, Sum/2, Mux/1, Scope13/1  "t_FL"
  CAN Unpack1/4 -> Mux/2  "t_FR"
  CAN Unpack3/4 -> Mux/4  "t_RR"
  Mux/1 -> To File/1, Scope7/1
  CAN Unpack4/1 -> To File1/1, testTs/1, Scope9/1
  CAN Unpack4/2 -> Scope10/1
  Sum/1 -> Scope11/1, timestampFL/1
  Memory/1 -> Sum/1
  CAN Unpack5/1 -> Gain/1
  Mux1/1 -> To File2/1, CAN_SR/1
  CAN Unpack5/2 -> Gain1/1
  CAN Unpack5/3 -> Gain2/1
  CAN Unpack5/4 -> Gain3/1
  Gain/1 -> Mux1/1
  Gain1/1 -> Mux1/2
  Gain2/1 -> Mux1/3
  Gain3/1 -> Mux1/4
  CAN Unpack6/1 -> Scope15/1, Gain4/1
  Gain4/1 -> yawRateref/1, To File3/1

== system TV2016_CAN/CarMaker/IPG Vehicle1 ==
  Sync_In : Inport
  Vhcl.Model.Source : Inport  Port=2
  VhclCtrl.Steering : Inport  Port=3
  Vhcl.Wheel.In : Inport  Port=4
  Vhcl.Misc : Inport  Port=5
  VhclCtrl.Brake : Inport  Port=6
  VhclCtrl.PT : Inport  Port=7
  Brake : Subsystem
  CarAndTrailer : Subsystem
  PowerTrain : Subsystem
  Stop Simulation : Stop
  VehicleSource_BuiltIn : simulink/Logic and Bit Operations/Compare To Constant  relop=~=  const=1  OutDataTypeStr=boolean  ZeroCross=off
  Sync_Out : Outport
  wires:
  VhclCtrl.PT/1 -> PowerTrain/3(VhclCtrl.PT)
  Brake/1(Sync_Out) -> PowerTrain/1(Sync_In)
  CarAndTrailer/1(Sync_Out) -> Brake/1(Sync_In)
  CarAndTrailer/2(Brake.IF.In) -> Brake/2(Brake.IF.In)
  VhclCtrl.Brake/1 -> Brake/3(VhclCtrl.Brake)
  PowerTrain/1(Sync_Out) -> Sync_Out/1
  Vhcl.Misc/1 -> CarAndTrailer/4(Vhcl.Misc)
  Vhcl.Wheel.In/1 -> CarAndTrailer/3(Vhcl.Wheel.In)
  VhclCtrl.Steering/1 -> CarAndTrailer/2(VhclCtrl.Steering)
  Sync_In/1 -> CarAndTrailer/1(Sync_In)
  Vhcl.Model.Source/1 -> VehicleSource_BuiltIn/1
  VehicleSource_BuiltIn/1 -> Stop Simulation/1
  Brake/2(Vhcl.Wheel.PT) -> PowerTrain/2(Vhcl.Wheel.PT)

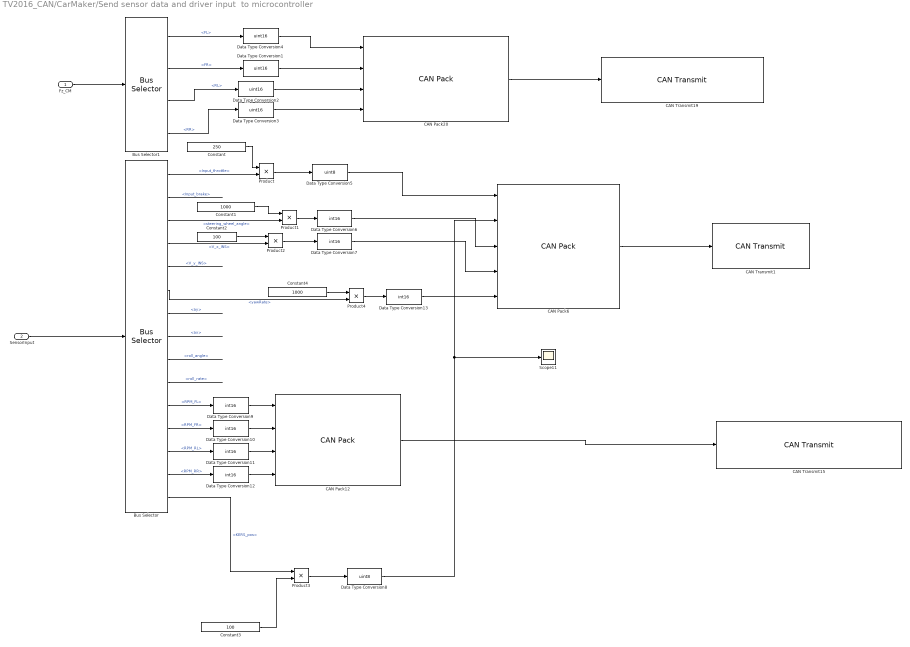
== system TV2016_CAN/CarMaker/Send sensor data and driver input  to microcontroller  ==
  Fz_CM : Inport
  SensorInput : Inport  Port=2
  Bus Selector : BusSelector  OutputSignals=Input_throttle,Input_brake,steering_wheel_angle,V_x_INS,V_y_INS,yawRate,ay,ax,roll_angle,roll_rate,RPM_FL,RPM_FR,RPM_RL,RPM_RR,KERS_pos
  Bus Selector1 : BusSelector  OutputSignals=FL,FR,RL,RR
  CAN Pack12 : canmsglib/CAN Pack  MsgList=(none)  MsgName=RPM  MsgIDType=Standard (11-bit identifier)  MsgIdentifier=502  MsgLength=8  SignalInfo=RPM_FL$0$16$1$1$1$0$1$0$-Inf$Inf$#RPM_FR$16$16$1$1$1$0$1$0$-Inf$Inf$#RPM_RL$32$16$1$1$1$0$1$0$-Inf$Inf$#RPM_RR$48$16$1$1$1$0$1$0$-Inf$Inf$#  NSignals=4  StartBits=str2num('[int32(0);int32(16);int32(32);int32(48)]')  SignalSizes=str2num('[int32(16);int32(16);int32(16);int32(16)]')  ByteOrders=str2num('[int32(1);int32(1);int32(1);int32(1)]')  DataTypes=str2num('[int32(1);int32(1);int32(1);int32(1)]')  MultiplexTypes=str2num('[int32(1);int32(1);int32(1);int32(1)]')  MultiplexValues=str2num('[double(0);double(0);double(0);double(0)]')  Factors=str2num('[double(1);double(1);double(1);double(1)]')  Offsets=str2num('[double(0);double(0);double(0);double(0)]')  Minimums=str2num('[double(-Inf);double(-Inf);double(-Inf);double(-Inf)]')  Maximums=str2num('[double(Inf);double(Inf);double(Inf);double(Inf)]')  Remote=off
      settings: DataFormat=manually specified signals
  CAN Pack20 : canmsglib/CAN Pack  MsgList=(none)  MsgName=Fz  MsgIDType=Standard (11-bit identifier)  MsgIdentifier=500  MsgLength=8  SignalInfo=Fz_FL$0$16$1$2$1$0$1$0$-Inf$Inf$#Fz_FR$16$16$1$2$1$0$1$0$-Inf$Inf$#Fz_RL$32$16$1$2$1$0$1$0$-Inf$Inf$#Fz_RR$48$16$1$2$1$0$1$0$-Inf$Inf$#  NSignals=4  StartBits=str2num('[int32(0);int32(16);int32(32);int32(48)]')  SignalSizes=str2num('[int32(16);int32(16);int32(16);int32(16)]')  ByteOrders=str2num('[int32(1);int32(1);int32(1);int32(1)]')  DataTypes=str2num('[int32(2);int32(2);int32(2);int32(2)]')  MultiplexTypes=str2num('[int32(1);int32(1);int32(1);int32(1)]')  MultiplexValues=str2num('[double(0);double(0);double(0);double(0)]')  Factors=str2num('[double(1);double(1);double(1);double(1)]')  Offsets=str2num('[double(0);double(0);double(0);double(0)]')  Minimums=str2num('[double(-Inf);double(-Inf);double(-Inf);double(-Inf)]')  Maximums=str2num('[double(Inf);double(Inf);double(Inf);double(Inf)]')  Remote=off
      settings: DataFormat=manually specified signals
  CAN Pack6 : canmsglib/CAN Pack  MsgList=(none)  MsgName=Senors  MsgIDType=Standard (11-bit identifier)  MsgIdentifier=501  MsgLength=8  SignalInfo=gas$0$8$1$2$1$0$1$0$-Inf$Inf$#kers$8$8$1$2$1$0$1$0$-Inf$Inf$#steering$16$16$1$1$1$0$1$0$-Inf$Inf$#vx$32$16$1$1$1$0$1$0$-Inf$Inf$#yawrate$48$16$1$1$1$0$1$0$-Inf$Inf$#  NSignals=5  StartBits=str2num('[int32(0);int32(8);int32(16);int32(32);int32(48)]')  SignalSizes=str2num('[int32(8);int32(8);int32(16);int32(16);int32(16)]')  ByteOrders=str2num('[int32(1);int32(1);int32(1);int32(1);int32(1)]')  DataTypes=str2num('[int32(2);int32(2);int32(1);int32(1);int32(1)]')  MultiplexTypes=str2num('[int32(1);int32(1);int32(1);int32(1);int32(1)]')  MultiplexValues=str2num('[double(0);double(0);double(0);double(0);double(0)]')  Factors=str2num('[double(1);double(1);double(1);double(1);double(1)]')  Offsets=str2num('[double(0);double(0);double(0);double(0);double(0)]')  Minimums=str2num('[double(-Inf);double(-Inf);double(-Inf);double(-Inf);double(-Inf)]')  Maximums=str2num('[double(Inf);double(Inf);double(Inf);double(Inf);double(Inf)]')  Remote=off
      settings: DataFormat=manually specified signals
  CAN Transmit1 : canlib/CAN Transmit  BlockHandle=12586.0002  DeviceMenu=(none)  Device=PEAK-System PCAN-USB (PCAN_USBBUS1)  ObjConstructor=canChannel('PEAK-System', 'PCAN_USBBUS1')  EnablePeriodicTransmit=on  MessagePeriod=0.01
  CAN Transmit15 : canlib/CAN Transmit  BlockHandle=12587.0002  DeviceMenu=(none)  Device=PEAK-System PCAN-USB (PCAN_USBBUS1)  ObjConstructor=canChannel('PEAK-System', 'PCAN_USBBUS1')  EnablePeriodicTransmit=on  MessagePeriod=0.01
  CAN Transmit19 : canlib/CAN Transmit  BlockHandle=12588.0002  DeviceMenu=(none)  Device=PEAK-System PCAN-USB (PCAN_USBBUS1)  ObjConstructor=canChannel('PEAK-System', 'PCAN_USBBUS1')  EnablePeriodicTransmit=on  MessagePeriod=0.01
  Constant : Constant  Value=250
  Constant1 : Constant  Value=1000
  Constant2 : Constant  Value=100
  Constant3 : Constant  Value=100
  Constant4 : Constant  Value=1000
  Data Type Conversion{1..4} (4 alike) : DataTypeConversion  OutDataTypeStr=uint16
  Data Type Conversion{6..7,9..13} (7 alike) : DataTypeConversion  OutDataTypeStr=int16
  Data Type Conversion5 : DataTypeConversion  OutDataTypeStr=uint8
  Data Type Conversion8 : DataTypeConversion  OutDataTypeStr=uint8
  Product{,1..4} (5 alike) : Product
  Scope11 : Scope
      settings: ShowLegends=on  TimeRange=2.184524711696869  YMin=-0.01  YMax=0.02  SaveName=ScopeData32
  wires:
  SensorInput/1 -> Bus Selector/1
  Bus Selector/2 -> ?  "<Input_brake>"
  Bus Selector/3 -> Product1/2  "<steering_wheel_angle>"
  Bus Selector/5 -> ?  "<V_y_INS>"
  Bus Selector/6 -> Product4/2  "<yawRate>"
  Bus Selector/7 -> ?  "<ay>"
  Bus Selector/8 -> ?  "<ax>"
  Bus Selector/9 -> ?  "<roll_angle>"
  Bus Selector/10 -> ?  "<roll_rate>"
  Bus Selector/11 -> Data Type Conversion9/1  "<RPM_FL>"
  Bus Selector/12 -> Data Type Conversion10/1  "<RPM_FR>"
  Bus Selector/13 -> Data Type Conversion11/1  "<RPM_RL>"
  Bus Selector/14 -> Data Type Conversion12/1  "<RPM_RR>"
  Fz_CM/1 -> Bus Selector1/1
  Bus Selector1/1 -> Data Type Conversion4/1  "<FL>"
  Bus Selector1/2 -> Data Type Conversion1/1  "<FR>"
  Bus Selector1/4 -> Data Type Conversion3/1  "<RR>"
  Bus Selector1/3 -> Data Type Conversion2/1  "<RL>"
  CAN Pack20/1 -> CAN Transmit19/1
  CAN Pack6/1 -> CAN Transmit1/1
  Data Type Conversion4/1 -> CAN Pack20/1
  Data Type Conversion1/1 -> CAN Pack20/2
  Data Type Conversion2/1 -> CAN Pack20/3
  Data Type Conversion3/1 -> CAN Pack20/4
  Bus Selector/1 -> Product/2  "<Input_throttle>"
  Constant/1 -> Product/1
  Product/1 -> Data Type Conversion5/1
  Data Type Conversion5/1 -> CAN Pack6/1
  Constant1/1 -> Product1/1
  Product1/1 -> Data Type Conversion6/1
  Data Type Conversion6/1 -> CAN Pack6/3
  Bus Selector/4 -> Product2/2  "<V_x_INS>"
  Constant2/1 -> Product2/1
  Product2/1 -> Data Type Conversion7/1
  Data Type Conversion7/1 -> CAN Pack6/4
  Constant3/1 -> Product3/2
  Product3/1 -> Data Type Conversion8/1
  Bus Selector/15 -> Product3/1  "<KERS_pos>"
  Data Type Conversion8/1 -> CAN Pack6/2, Scope11/1
  CAN Pack12/1 -> CAN Transmit15/1
  Data Type Conversion9/1 -> CAN Pack12/1
  Data Type Conversion10/1 -> CAN Pack12/2
  Data Type Conversion11/1 -> CAN Pack12/3
  Data Type Conversion12/1 -> CAN Pack12/4
  Product4/1 -> Data Type Conversion13/1
  Data Type Conversion13/1 -> CAN Pack6/5
  Constant4/1 -> Product4/1
